simulink model "env"  (R2024b)
settings: Solver=VariableStepAuto  StartTime=0.0  StopTime=1000  RelTol=1e-3  AbsTol=1e-3  EnableMultiTasking=on
PreLoadFcn:
  | inertiaDriveShaft = 12;
  | ratioDiff = 2;
  | radiusWheel = 16*2.54/100;
  | massVehicle = 1500;
  | inertiaLateral = 25*(radiusWheel)^2;
  | beta = 15;
  | engineRPM0 = 800;
  | tireStiffness = 200000;
  | tireDamping = 1000;
  | 
  | Simple=Simulink.VariantExpression('TIRE==1');
  | Friction=Simulink.VariantExpression('TIRE==2');
  | MFormula=Simulink.VariantExpression('TIRE==3');
  | 
  | TIRE=3;
model workspace (MAT data in the model file):
  Beta = -10
  Toque1 = 0
  Toque_f = 0
  Toque_r = 100
  Torque_f = 0
  Torque_r = 0
libraries: sdl_lib x18, nesl_utility x10, fl_lib x4, fl_ps_legacy_lib x4
(part 1 of 6)
CloseFcn:
  | try,close(h1_VehicleWithFourWheelDrive),end
  | clear h1_VehicleWithFourWheelDrive
  | 
  | 
  | clear simlog_VehicleWithFourWheelDrive
Description:
  | Vehicle with Four-Wheel Drive
settings Model: Creator=The MathWorks, Inc.  LastModifiedBy=23607
settings SolverCC: AutoScaleAbsTol=off  ZcThreshold=0  MaxConsecutiveMinStep=10  ZeroCrossAlgorithm=Adaptive  AlgebraicLoopSolver=TrustRegion
settings DataIOCC: LimitDataPoints=on  MaxDataPoints=10000  SaveFormat=Array  ReturnWorkspaceOutputs=off  SignalLoggingName=logsout_VehicleWithFourWheelDrive
settings OptimizationCC: ExpressionDepthLimit=2147483647  InitFltsAndDblsToZero=on  LifeSpan=inf  BufferReusableBoundary=off
settings DebuggingCC: SaveWithParameterizedLinksMsg=none  SignalResolutionControl=TryResolveAllWithWarning  MultiTaskDSMMsg=warning  MultiTaskCondExecSysMsg=none  SigSpecEnsureSampleTimeMsg=none  UnconnectedInputMsg=warning  UnconnectedOutputMsg=warning  UnconnectedLineMsg=warning  BusObjectLabelMismatch=none  StateNameClashWarn=warning  PregeneratedLibrarySubsystemCodeDiagnostic=none  SFUnexpectedBacktrackingDiag=warning  SFNoUnconditionalDefaultTransitionDiag=warning  SFExecutionAtInitializationDiag=none  ArithmeticOperatorsInVariantConditions=warning
settings HardwareCC: ProdBitPerPointer=32  ProdBitPerSizeT=32  ProdBitPerPtrDiffT=32  ProdLargestAtomicFloat=None  ProdIntDivRoundTo=Undefined  ProdEndianess=Unspecified  ProdWordSize=32  ProdHWDeviceType=32-bit Generic  TargetBitPerPointer=64  TargetBitPerSizeT=64  TargetBitPerPtrDiffT=64  TargetLongLongMode=on  TargetIntDivRoundTo=Zero  TargetEndianess=LittleEndian  TargetWordSize=64  TargetHWDeviceType=MATLAB Host  ProdEqTarget=off
settings ModelReferenceCC: EnableRefExpFcnMdlSchedulingChecks=on  PropagateSignalLabelsOutOfModel=off
settings SFSimCC: SimUseLocalCustomCode=off  CustomCodeUndefinedFunction=UseInterfaceOnly
settings RTWCC: RTWUseLocalCustomCode=off  GPUComputeCapability=3.5  DLArmComputeVersion=19.05
settings CodeAppCC: StateflowObjectComments=on
settings GRTTargetCC: TargetLangStandard=C89/C90 (ANSI)  CombineOutputUpdateFcns=off  GRTInterface=on
settings ConfigComp: CovMetricSettings=dw  CovSaveCumulativeToWorkspaceVar=on  CovSaveSingleToWorkspaceVar=on  CovExternalEMLEnable=off  CovSFcnEnable=off
settings SimscapeCC: SimscapeLogType=all  SimscapeLogSimulationStatistics=on  SimscapeLogName=simlog_VehicleWithFourWheelDrive  SimscapeLogDataHistory=15000

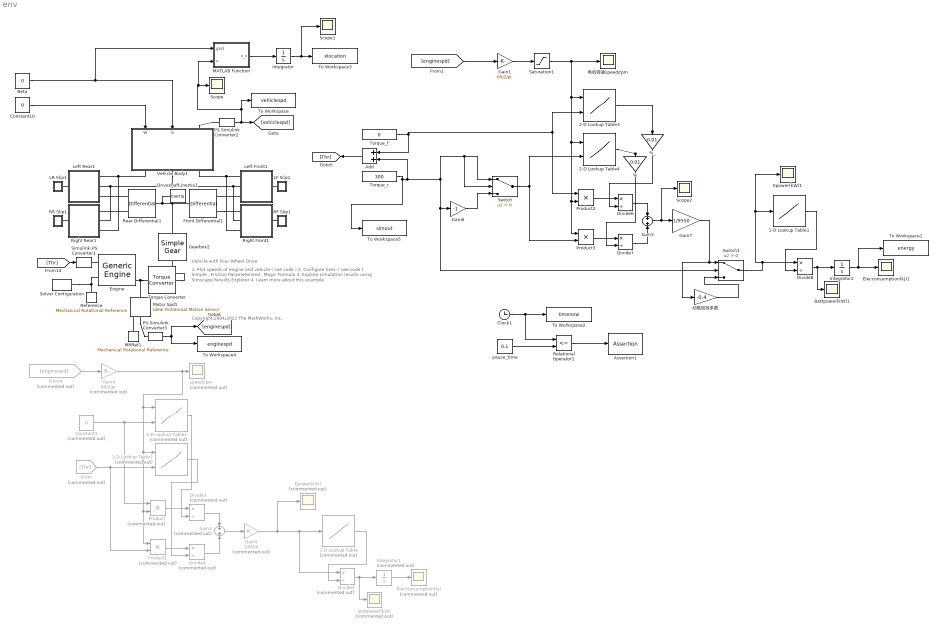
== system env ==
  note: Vehicle with Four-Wheel Drive
  note: 1. Plot speeds of engine and vehicle ( see code )
      | 2. Configure tires: ( see code )
      | Simple , Friction Parameterized , Magic Formula
      | 3. Explore simulation results using Simscape Results Explorer
      | 4. Learn more about this example
  note: Copyright 2004-2022 The MathWorks, Inc.
  % : Gain  Gain=0.01
  %_ : Gain  Gain=0.01
  1-D Lookup Table : Lookup_n-D  Commented=on  NumberOfTableDimensions=1  BreakpointsForDimension1=[0:10:100]  Table=[80 90 95 95 95 92 88 85 83 80 78]  InternalRulePriority=Speed  RndMeth=Simplest
  1-D Lookup Table1 : Lookup_n-D  NumberOfTableDimensions=1  BreakpointsForDimension1=[0:10:100]  Table=[0.80 0.90 0.95 0.95 0.95 0.92 0.88 0.85 0.83 0.80 0.78]  InternalRulePriority=Speed  RndMeth=Simplest
  2-D Lookup Table1 : Lookup_n-D  Commented=on  BreakpointsForDimension1=[0:1000:7000]  BreakpointsForDimension2=[0:50:350]  Table=[50 60 70 80 90 88 85 80;70 90 95 95.5 95 93 88 85;80 92.5 95 96 95 94 90 70;75 90 93 95 92 85 70 50;50 85 90 85 75 40 35 30;45 80 85 80 60 30 20 10;30 80 70 30 30 30 10 10;20 75 20 20 20 20 10 10]  InternalRulePriority=Speed  RndMeth=Simplest
      settings: InputPortMap=u0,u1
  2-D Lookup Table2 : Lookup_n-D  Commented=on  BreakpointsForDimension1=[0:1000:7000]  BreakpointsForDimension2=[0:50:350]  Table=[50 60 70 80 90 88 85 80;70 90 95 95.5 95 93 88 85;80 92.5 95 96 95 94 90 70;75 90 93 95 92 85 70 50;50 85 90 85 75 40 35 30;45 80 85 80 60 30 20 10;30 80 70 30 30 30 10 10;20 75 20 20 20 20 10 10]  InternalRulePriority=Speed  RndMeth=Simplest
      settings: InputPortMap=u0,u1
  2-D Lookup Table3 : Lookup_n-D  BreakpointsForDimension1=[0:1000:7000]  BreakpointsForDimension2=[0:50:350]  Table=[50 60 70 80 90 88 85 80;70 90 95 95.5 95 93 88 85;80 92.5 95 96 95 94 90 70;75 90 93 95 92 85 70 50;50 85 90 85 75 40 35 30;45 80 85 80 60 30 20 10;30 80 70 30 30 30 10 10;20 75 20 20 20 20 10 10]  InternalRulePriority=Speed  RndMeth=Simplest
      settings: InputPortMap=u0,u1
  2-D Lookup Table4 : Lookup_n-D  BreakpointsForDimension1=[0:1000:7000]  BreakpointsForDimension2=[0:50:350]  Table=[50 60 70 80 90 88 85 80;70 90 95 95.5 95 93 88 85;80 92.5 95 96 95 94 90 70;75 90 93 95 92 85 70 50;50 85 90 85 75 40 35 30;45 80 85 80 60 30 20 10;30 80 70 30 30 30 10 10;20 75 20 20 20 20 10 10]  InternalRulePriority=Speed  RndMeth=Simplest
      settings: InputPortMap=u0,u1
  Add : Sum
  Assertion1 : Assertion  AssertionFailFcn=set_param(bdroot, 'SimulationCommand', 'pause')  StopWhenAssertionFail=off
  Battpower(kW) : Scope  Commented=on
  Battpower(kW)1 : Scope
  Beta : Constant  Value=0
  Clock1 : Clock
  Constant10 : Constant  Value=0
  Constant3 : Constant  Commented=on  Value=0
  Divide3 : Product  Commented=on  Inputs=*/
  Divide4 : Product  Commented=on  Inputs=*/
  Divide5 : Product  Commented=on  Inputs=*/
  Divide6 : Product  Inputs=*/
  Divide7 : Product  Inputs=*/
  Divide8 : Product  Inputs=*/
  Driveshaft Inertia1 : fl_lib/Mechanical/Rotational Elements/Inertia  inertia=inertiaDriveShaft kg*m^2  num_ports=foundation.enum.numPorts2.one  w_specify=on  w_priority=None  w=0 rpm  w_nominal_specify=off  w_nominal_value=1  w_nominal_unit=rad/s  t_specify=off  t_priority=High  t=0 N*m  t_nominal_specify=off  t_nominal_value=1  t_nominal_unit=N*m
  Elecconsumption(kJ) : Scope  Commented=on
  Elecconsumption(kJ)1 : Scope
  Engine : sdl_lib/Engines & Motors/Generic Engine  input_type=sdl.enum.GenericEngineInputType.TorqueCommand  model_parameterization=1  engine_type=1  Trq_max=380 N*m  w_Trq_max=4300 rpm  P_max=150e3 W  w_P_max=4500 rpm  w_max=6000 rpm  w_min=500 rpm  w_tab=[ 500 1000 2e+3 3e+3 4e+3 5e+3 6e+3 7e+3 ] rpm  trq_tab=[ 380 380 380 380 350 280 200 80 ] N*m  pwr_tab=[ 2e+4 4e+4 7.8e+4 1.2e+5 1.45e+5 1.48e+5 1.25e+5 6e+4 ] W  interp_method=simscape.enum.interpolation.linear  w_thr=500 rpm  model_inertia=1  inertia=0.2 kg*m^2  initial_velocity=engineRPM0 rpm  model_time_constant=0  time_constant=0.2 s  initial_normalized_throttle=0  fc_model=0  fc_per_rev=25 mg/rev  fc_w_tab=[ 1000 2e+3 3e+3 4e+3 5e+3 6e+3 ] rpm  fc_trq_tab=[ 0 80 160 200 240 320 360 400 ] N*m  fc_tab=[ 0.5 0.9 1.4 1.6 1.9 2.7 3.4 4.4; 1 1.7 2.7 3.1 3.6 5 6 7.4; 1.4 2.7 4 4.8 5.6 7.5 8.5 10.5; 2 3.6 5.8 6.7 8 10.4 11.7 13.3; 2.5 4.8 7.9 9.4 10.8 14 16.2 18.6; 3.1 6 10.3 11.9 13.8 18.4 22 26.5 ] g/s  bmep_tab=[ 0 250 500 625 750 1000 1.15e+3 1.25e+3 ] kPa  bsfc_tab=[ 410 380 300 280 270 290 320 380; 410 370 290 270 260 270 285 320; 415 380 290 275 265 270 270 300; 420 390 310 290 285 280 280 285; 430 410 340 320 310 300 310 320; 450 430 370 340 330 330 350 380 ] g/hr/kW  fc_interp_method=simscape.enum.interpolation.linear  displaced_volume=400 cm^3  rev_per_cycle=2  idle_speed=0  idle_speed_reference=1000 rpm  tau_controller=1 s  idle_w_thr=1 rpm  redline=0  redline_speed=5000 rpm  tau_redline=1 s  redline_w_thr=1 rpm
      settings: InternalSimscapePortConfiguration="{\"Bottom\":[],\"Left\":[{\"id\":\"TrqCmd\",\"label\":\"Trq\",\"type\":\"input\"},{\"id\":\"B\",\"label\":\"B\",\"type\":\"foundation.mechanical.rotational.rotational\"}],\"Right\":[{\"id\":\"P\",\"label\":\"P\",\"type\":\"output\"},{\"id\":\"FC\",\"label\":\"FC\",\"type\":\"output\"},{\"id\":\"F\",\"label\":\"F\",\"type\":\"foundation.mechanical.rotational.rotational\"}],\"Top\":[]}"
  Epower(kW) : Scope  Commented=on
  Epower(kW)1 : Scope
  From : From  Commented=on  GotoTag=Thr
  From4 : From  Commented=on  GotoTag=enginespd
  Front Differential1 : sdl_lib/Gears/Differential  driveshaft_location=sdl.enum.differential_orientation.right  cd_ratio=(ratioDiff) * 2  friction_model=sdl.enum.gear_friction.none  efficiency=[ 0.85 0.92 ]  temperature_TLU=[ 280 300 320 ] K  efficiency_ss_TLU=[ 0.95 0.9 0.85 ]  efficiency_cd_TLU=[ 0.95 0.9 0.85 ]  pwr_thr=[ 0.001 0.001 ] W  mu_visc=[ 0 0 ] N*m/(rad/s)  model_inertia=1  sun_inertia=1e-10 kg*m^2  sun_radius=0.01 m  carrier_inertia=0.1 kg*m^2  planet_inertia=0.1 kg*m^2  planet_mass=1e-10 kg  thermal_mass=50 J/K  T_init=300 K
  Gain1 : Gain  Gain=60/2/pi
  Gain4 : Gain  Commented=on  Gain=60/2/pi
  Gain5 : Gain  Commented=on  Gain=1/9550
  Gain6 : Gain  Gain=-1
  Gain7 : Gain  Gain=1/9550
  Gearbox2 : sdl_lib/Gears/Simple Gear  ratio=2  rotation_direction=3-2*(1)  friction_model=1  T_noload=0.1 N*m  T_nom=5 N*m  efficiency_nom=0.8  efficiency=0.8  temperature_TLU=[ 280 300 320 ] K  load_TLU=[ 1 5 10 ] N*m  efficiency_TLU=[ 0.95 0.9 0.85 ]  efficiency_TLU2=[ 0.85 0.8 0.75; 0.95 0.9 0.85; 0.85 0.8 0.7 ]  w_thr=0.01 rad/s  pwr_thr=0.001 W  enable_backlash=false  hardstop_model=simscape.enum.hardstop.smooth  backlash_distance=1e-3 mm  r_base=0.1 m  transition=1e-4 mm  backlash_stiffness=1e7 N/m  backlash_damping=1e6 N*s/m  coeff_rest=0  v_tol=0.001 m/s  f_tol=0 N  mu_visc=[ 0 0 ] N*m/(rad/s)  thermal_mass=50 J/K  temperature_specify=off  temperature_priority=High  temperature=300 K  temperature_nominal_specify=off  temperature_nominal_value=1  temperature_nominal_unit=K  x_backlash_specify=off  x_backlash_priority=None  x_backlash=0 mm  x_backlash_nominal_specify=off  x_backlash_nominal_value=1  x_backlash_nominal_unit=mm  f_hardstop_specify=off  f_hardstop_priority=None  f_hardstop=0 N  f_hardstop_nominal_specify=off  f_hardstop_nominal_value=1  f_hardstop_nominal_unit=N  v_backlash_specify=off  v_backlash_priority=None  v_backlash=0 m/s  v_backlash_nominal_specify=off  v_backlash_nominal_value=1  v_backlash_nominal_unit=m/s
  Integrator : Integrator
  Integrator1 : Integrator  Commented=on
  Integrator2 : Integrator
  LF Slip1 : Subsystem
  LR Slip1 : Subsystem
  Left Front1 : Subsystem  Variant=on
      mask Display:
      | blk = get_param(gcb, 'CompiledActiveChoiceBlock');
      | eval(get_param(blk, 'MaskDisplay'));
  Left Rear1 : Subsystem  Variant=on
      mask Display:
      | blk = get_param(gcb, 'CompiledActiveChoiceBlock');
      | eval(get_param(blk, 'MaskDisplay'));
  MATLAB Function : MATLAB Function  TreatAsAtomicUnit=on
  MRRef1 : fl_lib/Mechanical/Rotational Elements/Mechanical Rotational Reference
  Motor Spd1 : fl_lib/Mechanical/Mechanical Sensors/Ideal Rotational Motion Sensor  reference=foundation.enum.MeasurementReference.difference  acceleration_port=false  velocity_port=true  position_port=true  wrap_angle=simscape.enum.onoff.off  offset=0 rad
      settings: LogSimulationData=on
  PS-Simulink Converter2 : nesl_utility/PS-Simulink Converter  PhysicalDomain=network_engine_domain  SubClassName=ps_output  LeftPortType=input  RightPortType=output  PseudoPeriodic=off  Frequencies=[]  VectorFormat=1-D array  Unit=m/s  AffineConversion=off
  PS-Simulink Converter3 : nesl_utility/PS-Simulink Converter  PhysicalDomain=network_engine_domain  SubClassName=ps_output  LeftPortType=input  RightPortType=output  PseudoPeriodic=off  Frequencies=[]  VectorFormat=1-D array  Unit=rad/s  AffineConversion=off
  Product : Product  Commented=on
  Product1 : Product  Commented=on
  Product2 : Product
  Product3 : Product
  RF Slip1 : Subsystem
  RR Slip1 : Subsystem
  Rear Differential1 : sdl_lib/Gears/Differential  driveshaft_location=sdl.enum.differential_orientation.right  cd_ratio=(ratioDiff) * 2  friction_model=sdl.enum.gear_friction.none  efficiency=[ 0.85 0.92 ]  temperature_TLU=[ 280 300 320 ] K  efficiency_ss_TLU=[ 0.95 0.9 0.85 ]  efficiency_cd_TLU=[ 0.95 0.9 0.85 ]  pwr_thr=[ 0.001 0.001 ] W  mu_visc=[ 0 0 ] N*m/(rad/s)  model_inertia=1  sun_inertia=1e-10 kg*m^2  sun_radius=0.01 m  carrier_inertia=0.1 kg*m^2  planet_inertia=0.1 kg*m^2  planet_mass=1e-10 kg  thermal_mass=50 J/K  T_init=300 K
  Reference : fl_lib/Mechanical/Rotational Elements/Mechanical Rotational Reference
  Relational Operator1 : RelationalOperator  Operator=<=  OutDataTypeStr=boolean  RndMeth=Simplest  InputSameDT=off
  Right Front1 : Subsystem  Variant=on
      settings: AttributesFormatString=%<ActiveVariant>
      mask Display:
      | blk = get_param(gcb, 'CompiledActiveChoiceBlock');
      | eval(get_param(blk, 'MaskDisplay'));
  Right Rear1 : Subsystem  Variant=on
      mask Display:
      | blk = get_param(gcb, 'CompiledActiveChoiceBlock');
      | eval(get_param(blk, 'MaskDisplay'));
  Saturation1 : Saturate  UpperLimit=5000  LowerLimit=0
  Scope : Scope
  Scope1 : Scope
  Scope2 : Scope
  Simulink-PS Converter1 : nesl_utility/Simulink-PS Converter  PhysicalDomain=network_engine_domain  SubClassName=ps_input  LeftPortType=input  RightPortType=output  PseudoPeriodic=off  Frequencies=[]  NoiseDistribution=none  NoiseParameters=[]  Unit=1  AffineConversion=off  FilteringAndDerivatives=zero  SimscapeFilterOrder=1  InputFilterTimeConstant=.001  UdotUserProvided=0
  Solver Configuration : nesl_utility/Solver Configuration  PhysicalDomain=network_engine_domain  SubClassName=solver  LeftPortType=input  RightPortType=generic  Tones=[]  Harmonics=[]  SimulateNoise=off  Profile=off  UseLocalSampling=off  EnableSwitchedLinearOptims=on  FrequencyDomain=off  UseCCode=off  RelTol=0.001  AbsTol=1e-06  MinStep=1e-09  ToWorkspace=off  RevertToSquareIcSolve=off  NumHomotopyIterations=100  PhasorMode=off  PhasorModeNumHarmonics=1  ConsistencySolver=NEWTON_XTOL_AFTER_FTOL  IndexReductionMethod=DerivativeReplacement  DoDC=off  ResidualTolerance=1e-9  ConsistencyTolSource=GLOBAL  ConsistencyAbsTol=0.001  ConsistencyRelTol=0.001  ConsistencyTolFactor=0.001  UseLocalSolver=off  LocalSolverChoice=NE_PARTITIONING_ADVANCER  ResolveIndetEquations=on  FunctionEvalNumThread=1  LocalSolverSampleTime=0.001  DoFixedCost=off  MaxNonlinIter=3  MaxModeIter=2  ComputeImpulses=off  ImpulseIterations=2  LinearAlgebra=auto  LinearAlgebraNumThread=0  EquationFormulation=NE_TIME_EF  DelaysMemoryBudget=1024  AutomaticFiltering=on  FilteringTimeConstant=0.001  PartitionStorageMethod=EXHAUSTIVE  PartitionMemoryBudget=1024  PartitionMethod=ROBUST  MultibodyUseLocalSolver=off  MultibodyLocalSolverChoice=ODE1  MultibodyLocalSolverSampleTime=0.001
  Sum2 : Sum  Commented=on  Inputs=+|+
  Sum3 : Sum  Inputs=+|+
  Switch : Switch  Criteria=u2 > Threshold  SaturateOnIntegerOverflow=off  InputSameDT=off
  Switch1 : Switch  Criteria=u2 > Threshold  SaturateOnIntegerOverflow=off  InputSameDT=off
  To Workspace : ToWorkspace  VariableName=vehiclespd  SampleTime=-1
  To Workspace1 : ToWorkspace  VariableName=energy  SampleTime=-1
  To Workspace2 : ToWorkspace  VariableName=timenow  SampleTime=0.1
  To Workspace3 : ToWorkspace  VariableName=xlocation  SampleTime=-1
  To Workspace4 : ToWorkspace  VariableName=enginespd  SampleTime=-1
  To Workspace5 : ToWorkspace  VariableName=simout  SampleTime=-1
  Torque Converter : sdl_lib/Couplings & Drives/Torque Converter  coast_mode_modeling=sdl.enum.torqueConverterContinuousTwomode.continuous  SR_drive_tlu=[0, .5, .6, .7, .8, .87, .92, .94, .96, .97, 1]  TR_drive_tlu=[2.232, 1.5462, 1.4058, 1.2746, 1.1528, 1.0732, 1.0192, 1, 1, 1, 1]  CF_drive_tlu=1e-4 * [.72558, .66322, .63463, .59042, .51331, .4144, .29287, .22444, .12186, .04386, 0] m*N/rpm^2  SR_coast_tlu=[0, .5, .6, .7, .8, .87, .92, .94, .96, .97, 1]  CF_coast_tlu=1e-4 * [.5079, .4643, .4442, .4133, .3593, .2901, .205, .1571, .0853, .0307, 0] m*N/rpm^2  iniMode=sdl.enum.torqueConverterInitialMode.drive  delta_w=1 rpm  n_vector=[0 0.50 0.60 0.70 0.80 0.87 0.92 0.94 0.96 0.97]  trq_vector=[2.2320 1.5462 1.4058 1.2746 1.1528 1.0732 1.0192 0.9983 0.9983 0.9983]  cf_vector_parameterization=1  cf_vector_reference_speed=1  cf_vector=[12.2938 12.8588 13.1452 13.6285 14.6163 16.2675 19.3503 22.1046 29.9986 50.00] (rad/s)/(N*m)^0.5  cf_vector_sq=1e-3*[ 6.616 6.048 5.787 5.384 4.681 3.779 2.671 2.047 1.111 0.400] N*m/(rad/s)^2  interp_method=1  extrap_method=1  model_lag=0  tau=0.02 s  initial_trq_ratio=0
      settings: InternalSimscapePortConfiguration="{\"Bottom\":[],\"Left\":[{\"id\":\"I\",\"label\":\"I\",\"type\":\"foundation.mechanical.rotational.rotational\"}],\"Right\":[{\"id\":\"T\",\"label\":\"T\",\"type\":\"foundation.mechanical.rotational.rotational\"}],\"Top\":[]}"
  Torque_f : Constant  Value=0
  Torque_r : Constant  Value=300
  Vehicle Body1 : Subsystem
      mask Display:
      | color('white')
      | plot(-120,-70); plot(120,40);
      | color('black')
      | plot(sin(0:0.1:6*pi)*15-70,cos(0:0.1:6*pi)*15-30);
      | plot(sin(0:0.1:6*pi)*15+70,cos(0:0.1:6*pi)*15-30);
      | plot([-88 -95 -99 -99 -95 -75 -65 -50 -46 10 30 34 80 85 90 93 95 93 90 88],[-30 -28 -23 -5 0 5 10 20 21 21 0 -2 -7 -9 -13 -17 -25 -28 -30 -30])
      | plot([-88 -95 -99 -99 -95 -75 -65 -50 -46 10 30 34 80 85 90 93 95 93 90 88],[-30 -28 -23 -5 0 5 10 20 21 21 0 -2 -7 -9 -13 -17 -25 -28 -30 -30]-1)
      | plot([-88 -95 -99 -99 -95 -75 -65 -50 -46 10 30 34 80 85 90 93 95 93 90 88]+1,[-30 -28 -23 -5 0 5 10 20 21 21 0 -2 -7 -9 -13 -17 -25 -28 -30 -30])
      | plot([-50 50],[-30 -30])
  pause_time : Constant  Value=0.1
  speed/rpm : Scope  Commented=on
  动能回收系数 : Gain  Gain=-0.4
  电机转速speed/rpm : Scope
  wires:
  Clock1/1 -> To Workspace2/1, Relational Operator1/1
  pause_time/1 -> Relational Operator1/2
  Relational Operator1/1 -> Assertion1/1
  2-D Lookup Table4/1 -> %/1
  Switch1/1 -> Epower(kW)1/1, 1-D Lookup Table1/1, Divide8/1
  Gain7/1 -> 动能回收系数/1, Switch1/1
  动能回收系数/1 -> Switch1/3
  Product2/1 -> Divide6/1
  Torque_r/1 -> To Workspace5/1, Add/2, Switch/2, Switch/1, Switch1/2, Gain6/1
  1-D Lookup Table1/1 -> Divide8/2
  Torque_f/1 -> 2-D Lookup Table3/2, Product2/1, Add/1
  2-D Lookup Table3/1 -> %_/1
  Divide8/1 -> Integrator2/1, Battpower(kW)1/1
  Product3/1 -> Divide7/1
  Gain6/1 -> Switch/3
  Divide7/1 -> Sum3/2
  Integrator2/1 -> To Workspace1/1, Elecconsumption(kJ)1/1
  Sum3/1 -> Scope2/1, Gain7/1
  Switch/1 -> Product3/2, 2-D Lookup Table4/2
  %_/1 -> Divide6/2
  Divide6/1 -> Sum3/1
  %/1 -> Divide7/2
  Beta/1 -> Vehicle Body1/2(b), MATLAB Function/1(grid)
  [Thr] -> Simulink-PS Converter1/1
  Constant10/1 -> Vehicle Body1/1(W)
  PS-Simulink Converter3/1 -> [enginespd], To Workspace4/1
  Gain1/1 -> Saturation1/1
  Constant3/1 -> Product/1, 2-D Lookup Table1/2
  From/1 -> Product1/2, 2-D Lookup Table2/2
  Gain4/1 -> Product/2, Product1/1, 2-D Lookup Table2/1, 2-D Lookup Table1/1, speed/rpm/1
  Divide5/1 -> Integrator1/1, Battpower(kW)/1
  Product/1 -> Divide3/1
  Gain5/1 -> Divide5/1, 1-D Lookup Table/1, Epower(kW)/1
  From4/1 -> Gain4/1
  Divide3/1 -> Sum2/1
  Divide4/1 -> Sum2/2
  Sum2/1 -> Gain5/1
  1-D Lookup Table/1 -> Divide5/2
  2-D Lookup Table2/1 -> Divide4/2
  2-D Lookup Table1/1 -> Divide3/2
  Product1/1 -> Divide4/1
  Integrator1/1 -> Elecconsumption(kJ)/1
  [enginespd] -> Gain1/1
  Saturation1/1 -> 电机转速speed/rpm/1, 2-D Lookup Table3/1, Product2/2, Product3/1, 2-D Lookup Table4/1
  Add/1 -> [Thr]
  Integrator/1 -> Scope1/1, To Workspace3/1
  PS-Simulink Converter2/1 -> To Workspace/1, MATLAB Function/2(v), Scope/1, [vehiclespd]
  MATLAB Function/1(v_x) -> Integrator/1
  connections:
  Left Front1/LConn2 -- Vehicle Body1/RConn2 -- Right Rear1/LConn2 -- Left Rear1/LConn2 -- Right Front1/LConn2
  Right Rear1/LConn1 -- Vehicle Body1/RConn1 -- Left Rear1/LConn1
  Right Front1/LConn1 -- Left Front1/LConn1 -- Vehicle Body1/RConn3
  Rear Differential1/LConn1 -- Gearbox2/RConn1 -- Front Differential1/LConn1 -- Driveshaft Inertia1/LConn1
  Engine/LConn2 -- Reference/LConn1 -- Solver Configuration/RConn1
  RF Slip1/LConn1 -- Right Front1/RConn1
  PS-Simulink Converter2/LConn1 -- Vehicle Body1/LConn1
  RR Slip1/LConn1 -- Right Rear1/RConn1
  Rear Differential1/RConn1 -- Left Rear1/LConn3
  Simulink-PS Converter1/RConn1 -- Engine/LConn1
  Left Front1/RConn1 -- LF Slip1/LConn1
  Torque Converter/RConn1 -- Gearbox2/LConn1
  Left Rear1/RConn1 -- LR Slip1/LConn1
  Rear Differential1/RConn2 -- Right Rear1/LConn3
  Left Front1/LConn3 -- Front Differential1/RConn1
  Front Differential1/RConn2 -- Right Front1/LConn3
  Engine/RConn3 -- Torque Converter/LConn1 -- Motor Spd1/LConn1
  Motor Spd1/RConn2 -- PS-Simulink Converter3/LConn1
  MRRef1/LConn1 -- Motor Spd1/RConn1

== system env/LF Slip1 ==
  PS-Simulink Converter : nesl_utility/PS-Simulink Converter  PhysicalDomain=network_engine_domain  SubClassName=ps_output  LeftPortType=input  RightPortType=output  PseudoPeriodic=off  Frequencies=[]  VectorFormat=1-D array  Unit=1  AffineConversion=off
  Terminator : Terminator
  S : PMIOPort  Side=Left
  wires:
  PS-Simulink Converter/1 -> Terminator/1
  connections:
  S/RConn1 -- PS-Simulink Converter/LConn1

== system env/LR Slip1 ==
  PS-Simulink Converter : nesl_utility/PS-Simulink Converter  PhysicalDomain=network_engine_domain  SubClassName=ps_output  LeftPortType=input  RightPortType=output  PseudoPeriodic=off  Frequencies=[]  VectorFormat=1-D array  Unit=1  AffineConversion=off
  Terminator : Terminator
  S : PMIOPort  Side=Left
  wires:
  PS-Simulink Converter/1 -> Terminator/1
  connections:
  S/RConn1 -- PS-Simulink Converter/LConn1
